simulink model "dsp48_firs_tb"  (Simulink 7.0)
settings: Solver=ode45  StartTime=0.0  StopTime=200  RelTol=1e-3
PreLoadFcn:
  | fir_setup_v1
StartFcn:
  | fir_setup_v1
undefined symbols (not defined in the file): A, B, C, coef, P, PCIN
libraries: xbsIndex_r4 x229, simulink x10, xbsCopyrightNotice_r4 x1, dspsrcs4 x1
(part 1 of 3)
settings Model: Creator=alexc  LastModifiedBy=douangp
settings DataIOCC: SignalLoggingName=sigsOut
settings OptimizationCC: InlineInvariantSignals=on
settings DebuggingCC: SaveWithParameterizedLinksMsg=none  SignalResolutionControl=TryResolveAllWithWarning  SolverPrmCheckMsg=none  MultiTaskDSMMsg=warning  MultiTaskCondExecSysMsg=none  StrictBusMsg=None
settings HardwareCC: TargetUnknown=on
settings RTWCC: IncludeERTFirstTime=on
settings GRTTargetCC: TargetFcnLib=ansi_tfl_tmw.mat

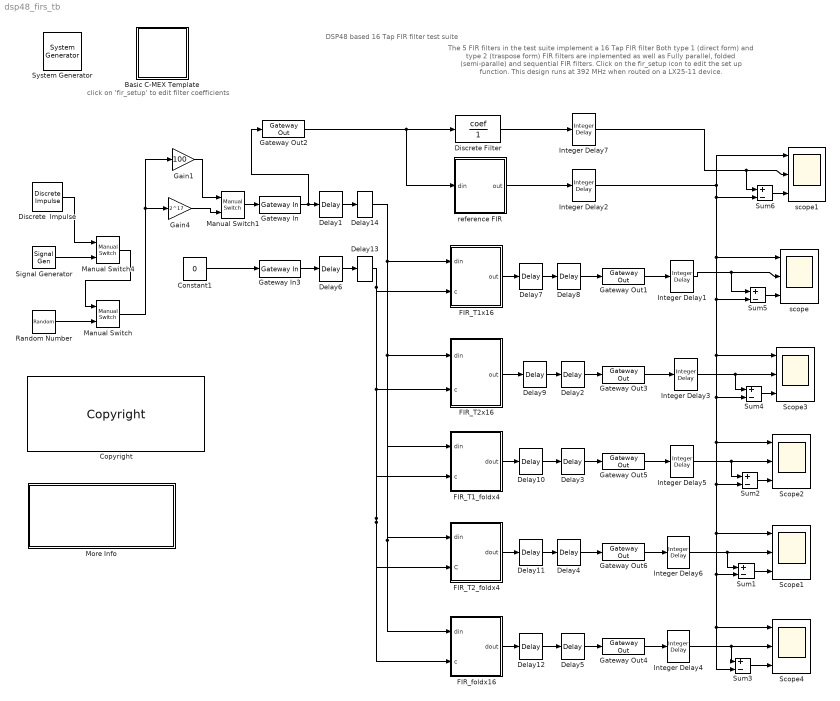
== system dsp48_firs_tb ==
  note: DSP48 based 16 Tap FIR filter test suite
  note: The 5 FIR filters in the test suite implement a 16 Tap FIR filter
      | Both type 1 (direct form) and type 2 (traspose form) FIR filters
      | are inplemented as well as Fully parallel, folded (semi-paralle)
      | and sequential FIR filters. Click on the fir_setup icon to edit the
      |  set up function.
      |
      | This design runs at 392 MHz when routed on a LX25-11 device.
  note: click on 'fir_setup'
      | to edit filter coefficients
  " System Generator" : xbsIndex_r4/ System Generator  Tag=genX  SystemSampleTime=-1  xilinxfamily=virtex4  part=xc4vlx25  speed=-11  package=ff668  synthesis_tool=XST  clock_wrapper=Clock Enables  directory=./netlist  testbench=off  simulink_period=1/16  sysclk_period=2.551  dcm_input_clock_period=100  incr_netlist=off  trim_vbits=Everywhere in SubSystem  dbl_ovrd=According to Block Masks  core_generation=According to Block Masks  run_coregen=off  deprecated_control=off  eval_field=0  block_type=system_generator
      settings: block_version=8.2.EA1
  "Basic C-MEX Template " : Subsystem  AncestorBlock=|
      | sfundemos/C-file
      | S-functions/Basic C-MEX
      | Template
      settings: OpenFcn=evalin('base','edit(''fir_setup_v1.m'')')
      mask Display:
      | plot([.8  0 0 1 1 .8 .8 1],[1 1 0 0 .7 .7 1 .7])
      | disp('fir_setup');
  Constant1 : Constant  Value=0  OutDataType=sfix(16)  OutScaling=2^0
  Copyright : xbsCopyrightNotice_r4/Copyright  block_type=copyright
      settings: block_version=10.1.00
      settings: infoedit=|
      | Copyright(C) 2008 by  Xilinx, Inc. All rights reserved.<br>
      | <br>
      | This file contains proprietary, confidential information of Xilinx, Inc., is distributed under license
      | from Xilinx, Inc., and may be used, copied and/or disclosed only pursuant to the terms of a valid license
      | agreement with Xilinx, Inc. Xilinx hereby grants you a license to use this file solely for design,
      | simulation, implementation and creation of design files limited to Xilinx devices or technologies. Use
      | with non-Xilinx devices or technologies is expressly prohibited and immediately terminates your license
      | unless covered by a separate agreement.<br>
      | <br>
      | Xilinx is providing this design, code, or information "as-is" solely for use in developing programs and
      | solutions for Xilinx devices, with no obligation on the part of Xilinx to provide support. By providing
      | this design, code, or information as one possible implementation of this feature, application or standard,
      | Xilinx is making no representation that this implementation is free from any claims of infringement. You
      | are responsible for obtaining any rights you may require for your implementation. Xilinx expressly disclaims
      | any warranty whatsoever with respect to the adequacy of the implementation, including but not limited to any
      | warranties or representations that this implementation is free from claims of infringement, implied warranties
      | of merchantability or fitness for a particular purpose.<br>
      | <br>
      | Xilinx products are not intended for use in life support appliances, devices, or systems. Use in such
      | applications is expressly prohibited.<br>
      | <br>
      | Any modifications that are made to the Source Code are done at the user's sole risk and will be unsupported.<br>
      | <br>
      | This copyright and support notice must be retained as part of this text at all times.
      | (c) Copyright 1995-2008 Xilinx, Inc. All rights reserved.
  Delay{1..14} (14 alike) : xbsIndex_r4/Delay  en=off  latency=1  dbl_ovrd=off  reg_retiming=off  block_type=delay
      settings: infoedit="Delay line having  configurable length.<P><P>Hardware notes: A delay line is a chain, each link of which is an SRL16 followed by a flip-flop. If register retiming is enabled, the delay line is a chain of flip-flops."  xl_area=[0, 0, 0, 0, 0, 0, 0]  block_version=VER_STRING_GOES_HERE
  Discrete  Impulse : dspsrcs4/Discrete  Impulse  Delay=0  SampleTime=1  FrameSample=1  dataType=double  isSigned=on  wordLen=16  udDataType=sfix(16)  fracBitsMode=Best precision  numFracBits=15
  Discrete Filter : DiscreteFilter  Numerator=coef  Denominator=1
  FIR_T1_foldx4 : Subsystem
  FIR_T1x16 : Subsystem
  FIR_T2_foldx4 : Subsystem
  "FIR_T2x16 " : Subsystem
  FIR_foldx16 : Subsystem
  Gain1 : Gain  Gain=100  ParameterDataType=sfix(16)  ParameterScaling=2^0  OutDataType=sfix(16)  OutScaling=2^0  SampleTime=1  SaturateOnIntegerOverflow=on
  Gain4 : Gain  Gain=2^17  ParameterDataType=sfix(16)  ParameterScaling=2^0  OutDataType=sfix(16)  OutScaling=2^0  SampleTime=1  SaturateOnIntegerOverflow=on
  Gateway In : xbsIndex_r4/Gateway In  arith_type="Signed  (2's comp)"  n_bits=18  bin_pt=0  quantization="Round  (unbiased: +/- Inf)"  overflow=Saturate  period=1  dbl_ovrd=off  timing_constraint=None  locs_specified=off  LOCs={}  block_type=gatewayin
      settings: infoedit="Gateway in block.  Converts inputs of type Simulink integer, double and fixed point to  Xilinx fixed point type.<P><P>Hardware notes:  In hardware these blocks become top level input ports."  xl_area=[0, 0, 0, 0, 0, 0, 0]  block_version=VER_STRING_GOES_HERE
  Gateway In3 : xbsIndex_r4/Gateway In  arith_type="Signed  (2's comp)"  n_bits=48  bin_pt=0  quantization="Round  (unbiased: +/- Inf)"  overflow=Saturate  period=1  dbl_ovrd=off  timing_constraint=None  locs_specified=off  LOCs={}  block_type=gatewayin
      settings: infoedit="Gateway in block.  Converts inputs of type Simulink integer, double and fixed point to  Xilinx fixed point type.<P><P>Hardware notes:  In hardware these blocks become top level input ports."  xl_area=[0, 0, 0, 0, 0, 0, 0]  block_version=VER_STRING_GOES_HERE
  Gateway Out{1..6} (6 alike) : xbsIndex_r4/Gateway Out  hdl_port=on  timing_constraint=None  locs_specified=off  LOCs={}  block_type=gatewayout
      settings: infoedit="Gateway out block.  Converts Xilinx fixed point inputs into ouputs of type Simulink integer, double, or fixed point.<P><P>Hardware notes:  In hardware these blocks become top level output ports or are discarded, depending on how they are configured."  xl_area=[0, 0, 0, 0, 0, 0, 0]  block_version=VER_STRING_GOES_HERE
  Integer Delay1 : simulink/Discrete/Integer Delay  vinit=0.0  samptime=-1  NumDelays=2
  Integer Delay2 : simulink/Discrete/Integer Delay  vinit=0.0  samptime=-1  NumDelays=25
  Integer Delay3 : simulink/Discrete/Integer Delay  vinit=0.0  samptime=-1  NumDelays=18
  Integer Delay4 : simulink/Discrete/Integer Delay  vinit=0.0  samptime=-1  NumDelays=17
  Integer Delay5 : simulink/Discrete/Integer Delay  vinit=0.0  samptime=-1  NumDelays=14
  Integer Delay6 : simulink/Discrete/Integer Delay  vinit=0.0  samptime=-1  NumDelays=12
  Integer Delay7 : simulink/Discrete/Integer Delay  vinit=0.0  samptime=-1  NumDelays=25
  Manual Switch : simulink/Signal Routing/Manual Switch  SystemSampleTime=-1  sw=0  action=0  varsize=off
  Manual Switch1 : simulink/Signal Routing/Manual Switch  SystemSampleTime=-1  sw=1  action=0  varsize=off
  Manual Switch4 : simulink/Signal Routing/Manual Switch  SystemSampleTime=-1  sw=1  action=0  varsize=off
  More Info : Subsystem
      settings: OpenFcn=xlDoc('-book','sysgen','-topic','Hardware Design Using System Generator/Design Styles for the DSP48/Designs that Use DSP48 and DSP48 Macro Blocks');
      mask Display: disp('Double click\n for System Generator\n documentation on related topics.')
  Random Number : RandomNumber  SampleTime=1
  Scope{1..4} (4 alike) : Scope  NumInputPorts=3
      Scope1 settings: TimeRange=200  YMin=-1e+007~-1e+007~-90  YMax=1e+007~1e+007~0
      Scope2 settings: TimeRange=200  YMin=129.2~105~105  YMax=142.8~140~140
      Scope3 settings: TimeRange=200  YMin=129.2~105~105  YMax=142.8~140~140  SaveName=ScopeData2
      Scope4 settings: TimeRange=200  YMin=-12500~-10000~950  YMax=7500~7000~1050  SaveName=ScopeData5
  Signal Generator : SignalGenerator  Frequency=.01
  Sum{1..6} (6 alike) : Sum  Inputs=+-  OutDataType=sfix(16)  OutScaling=2^0  SaturateOnIntegerOverflow=on
  reference FIR : Subsystem
  scope : Scope  NumInputPorts=3
      settings: TimeRange=200  YMin=-7500~-7500~-8000  YMax=12500~12500~7000  SaveName=ScopeData3
  scope1 : Scope  NumInputPorts=3
      settings: TimeRange=200  YMin=-12500~-12500~-1  YMax=7500~7500~1  SaveName=ScopeData4
  wires:
  Random Number/1 -> Manual Switch/2
  Gateway In/1 -> Delay1/1, Gateway Out2/1
  Constant1/1 -> Gateway In3/1
  Delay8/1 -> Gateway Out1/1
  Gateway Out1/1 -> Integer Delay1/1
  Delay2/1 -> Gateway Out3/1
  Gateway Out3/1 -> Integer Delay3/1
  Gateway Out5/1 -> Integer Delay5/1
  Gateway Out6/1 -> Integer Delay6/1
  Sum3/1 -> Scope4/3
  Manual Switch4/1 -> Manual Switch/1
  Signal Generator/1 -> Manual Switch4/2
  Discrete  Impulse/1 -> Manual Switch4/1
  FIR_T1_foldx4/1(dout) -> Delay10/1
  FIR_T2_foldx4/1(dout) -> Delay11/1
  FIR_foldx16/1(dout) -> Delay12/1
  Delay3/1 -> Gateway Out5/1
  Delay4/1 -> Gateway Out6/1
  Delay5/1 -> Gateway Out4/1
  Manual Switch/1 -> Gain4/1, Gain1/1
  Gateway In3/1 -> Delay6/1
  Delay1/1 -> Delay14/1
  Delay6/1 -> Delay13/1
  Integer Delay4/1 -> Scope4/2, Sum3/1
  Sum1/1 -> Scope1/3
  Integer Delay6/1 -> Sum1/1, Scope1/2
  Sum2/1 -> Scope2/3
  Integer Delay5/1 -> Scope2/2, Sum2/1
  Sum4/1 -> Scope3/3
  Integer Delay3/1 -> Sum4/1, Scope3/2
  Sum5/1 -> scope/3
  Integer Delay1/1 -> scope/2, Sum5/1
  reference FIR/1(out) -> Integer Delay2/1
  Integer Delay2/1 -> Scope3/1, Sum3/2, Scope4/1, Sum1/2, Scope1/1, Sum2/2, Scope2/1, Sum4/2, Sum5/2, scope/1, Sum6/2, scope1/1
  Manual Switch1/1 -> Gateway In/1
  Gain4/1 -> Manual Switch1/2
  Gain1/1 -> Manual Switch1/1
  Sum6/1 -> scope1/3
  Discrete Filter/1 -> Integer Delay7/1
  Integer Delay7/1 -> Sum6/1, scope1/2
  Gateway Out2/1 -> reference FIR/1(din), Discrete Filter/1
  Delay7/1 -> Delay8/1
  Delay9/1 -> Delay2/1
  Delay10/1 -> Delay3/1
  Delay11/1 -> Delay4/1
  Delay12/1 -> Delay5/1
  Delay13/1 -> FIR_T1_foldx4/2(c), FIR_T2_foldx4/2(C), FIR_foldx16/2(c), "FIR_T2x16 "/2(c), FIR_T1x16/2(c)
  Delay14/1 -> FIR_T1x16/1(din), FIR_T2_foldx4/1(din), FIR_T1_foldx4/1(din), FIR_foldx16/1(din), "FIR_T2x16 "/1(din)
  "FIR_T2x16 "/1(out) -> Delay9/1
  FIR_T1x16/1(out) -> Delay7/1
  Gateway Out4/1 -> Integer Delay4/1

== system dsp48_firs_tb/Basic C-MEX Template  ==
  "Basic C-MEX Template " : Subsystem  AncestorBlock=|
      | sfundemos/C-file
      | S-functions/Basic C-MEX
      | Template
      settings: OpenFcn=evalin('base','edit(''make_nio_io_cyc.m'')')
      mask Display:
      | plot([.8  0 0 1 1 .8 .8 1],[1 1 0 0 .7 .7 1 .7])
      | disp('make_nio_io_cyc.m');

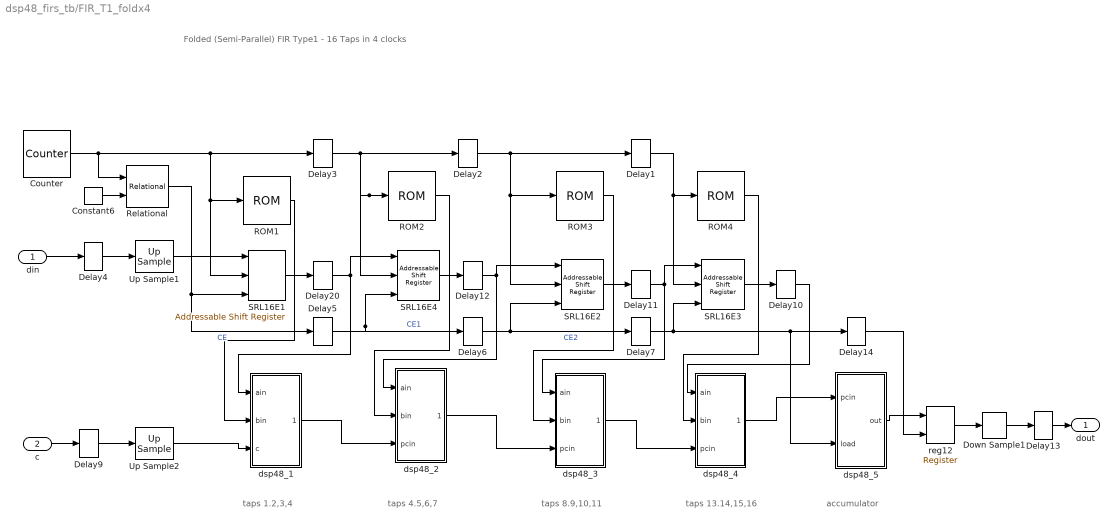
== system dsp48_firs_tb/FIR_T1_foldx4 ==
  note: Folded (Semi-Parallel) FIR Type1 - 16 Taps in 4 clocks
  note: taps 1.2,3,4
  note: taps 4.5,6,7
  note: taps 8.9,10,11
  note: taps 13.14,15,16
  note: accumulator
  din : Inport  OutDataType=sfix(16)  OutScaling=2^0
  c : Inport  Port=2  OutDataType=sfix(16)  OutScaling=2^0
  Constant6 : xbsIndex_r4/Constant  arith_type=Unsigned  const=3  n_bits=2  bin_pt=0  explicit_period=off  period=1  equ=P=C  opselect=C  inp2=PCIN>>17  opr=+  inp1=P  carry=CIN  dbl_ovrd=off  block_type=constant
      settings: block_version=VER_STRING_GOES_HERE
  Counter : xbsIndex_r4/Counter  cnt_type=Count Limited  cnt_to=3  operation=Up  start_count=0  cnt_by_val=1  arith_type=Unsigned  n_bits=2  bin_pt=0  load_pin=off  rst=off  en=off  explicit_period=off  period=1/4  dbl_ovrd=off  use_behavioral_HDL=off  use_rpm=off  block_type=counter
      settings: infoedit="Configurable up, down and up/down counter.<P><P>Hardware notes: Free running counters are the least expensive in hardware.  A count limited counter is implemented by combining a counter with a comparator."  xl_area=[2 2 0 3 0 0 0]  block_version=VER_STRING_GOES_HERE
  Delay{1..7,9..14,20} (14 alike) : xbsIndex_r4/Delay  en=off  latency=1  dbl_ovrd=off  reg_retiming=off  block_type=delay
      settings: infoedit="Delay line having  configurable length.<P><P>Hardware notes: A delay line is a chain, each link of which is an SRL16 followed by a flip-flop. If register retiming is enabled, the delay line is a chain of flip-flops."  xl_area=[0, 0, 0, 0, 0, 0, 0]  block_version=VER_STRING_GOES_HERE
  Down Sample1 : xbsIndex_r4/Down Sample  sample_ratio=4  sample_phase="Last Value of Frame  (most efficient)"  en=off  latency=1  dbl_ovrd=off  block_type=dsamp
      settings: xl_area=[24 48 0 0 0 0 0]  block_version=VER_STRING_GOES_HERE
  ROM1 : xbsIndex_r4/ROM  depth=4  initVector=coef(1:4)  distributed_mem=Distributed memory  rst=off  init_reg=0  en=off  latency=1  arith_type="Signed  (2's comp)"  n_bits=18  bin_pt=0  dbl_ovrd=off  optimize=Area  use_rpm=off  block_type=sprom
      settings: xl_area=[0, 0, 0, 0, 0, 0, 0]  block_version=VER_STRING_GOES_HERE
  ROM2 : xbsIndex_r4/ROM  depth=4  initVector=coef(5:8)  distributed_mem=Distributed memory  rst=off  init_reg=0  en=off  latency=1  arith_type="Signed  (2's comp)"  n_bits=18  bin_pt=0  dbl_ovrd=off  optimize=Area  use_rpm=off  block_type=sprom
      settings: xl_area=[0, 0, 0, 0, 0, 0, 0]  block_version=VER_STRING_GOES_HERE
  ROM3 : xbsIndex_r4/ROM  depth=4  initVector=coef(9:12)  distributed_mem=Distributed memory  rst=off  init_reg=0  en=off  latency=1  arith_type="Signed  (2's comp)"  n_bits=18  bin_pt=0  dbl_ovrd=off  optimize=Area  use_rpm=off  block_type=sprom
      settings: xl_area=[0, 0, 0, 0, 0, 0, 0]  block_version=VER_STRING_GOES_HERE
  ROM4 : xbsIndex_r4/ROM  depth=4  initVector=coef(13:16)  distributed_mem=Distributed memory  rst=off  init_reg=0  en=off  latency=1  arith_type="Signed  (2's comp)"  n_bits=18  bin_pt=0  dbl_ovrd=off  optimize=Area  use_rpm=off  block_type=sprom
      settings: xl_area=[0, 0, 0, 0, 0, 0, 0]  block_version=VER_STRING_GOES_HERE
  Relational : xbsIndex_r4/Relational  mode=a=b  en=off  latency=0  dbl_ovrd=off  block_type=relational
      settings: xl_area=[1 0 0 1 0 0 0]  block_version=VER_STRING_GOES_HERE
  SRL16E{1..4} (4 alike) : xbsIndex_r4/Addressable Shift Register  infer_latency=off  depth=4  initVector=[0]  en=on  dbl_ovrd=off  use_behavioral_HDL=off  use_rpm=off  block_type=addrsr
      settings: infoedit="Delay of configurable length.  Any element in the delay line can be addressed and driven onto the output port.<P><P>Hardware notes: Implemented using SRL16s.  If a Virtex-II device is used, multiple SRLC16s are cascaded together."  xl_area=[9 0 0 18 0 0 0]  block_version=VER_STRING_GOES_HERE
  Up Sample1 : xbsIndex_r4/Up Sample  sample_ratio=4  copy_samples=on  dbl_ovrd=off  block_type=usamp
      settings: infoedit="Up samples input data.  Inserted values  can be zeros or copies of the most recent input sample.<P><P>Hardware notes: No hardware is needed if inserted values are copies of the input sample; otherwise, a mux and single bit flip-flop are used."  xl_area=[0 0 0 0 0 0 0]  block_version=VER_STRING_GOES_HERE
  Up Sample2 : xbsIndex_r4/Up Sample  sample_ratio=4  copy_samples=on  dbl_ovrd=off  block_type=usamp
      settings: infoedit="Up samples input data.  Inserted values  can be zeros or copies of the most recent input sample.<P><P>Hardware notes: No hardware is needed if inserted values are copies of the input sample; otherwise, a mux and single bit flip-flop are used."  xl_area=[0 0 0 0 0 0 0]  block_version=VER_STRING_GOES_HERE
  dsp48_1 : Subsystem
  dsp48_2 : Subsystem
  dsp48_3 : Subsystem
  dsp48_4 : Subsystem
  dsp48_5 : Subsystem
  reg12 : xbsIndex_r4/Register  init=0  rst=off  en=on  dbl_ovrd=off  block_type=register
      settings: xl_area=[24 48 0 0 0 0 0]  block_version=VER_STRING_GOES_HERE
  dout : Outport  OutDataType=sfix(16)  OutScaling=2^0
  wires:
  SRL16E1/1 -> Delay20/1
  SRL16E4/1 -> Delay12/1
  ROM2/1 -> dsp48_2/2(bin)
  ROM1/1 -> dsp48_1/2(bin)
  ROM3/1 -> dsp48_3/2(bin)
  ROM4/1 -> dsp48_4/2(bin)
  dsp48_2/1(pcout) -> dsp48_3/3(pcin)
  dsp48_3/1(pcout) -> dsp48_4/3(pcin)
  SRL16E2/1 -> Delay11/1
  SRL16E3/1 -> Delay10/1
  Delay2/1 -> SRL16E2/2, ROM3/1, Delay1/1
  Delay1/1 -> SRL16E3/2, ROM4/1
  Delay12/1 -> SRL16E2/1, dsp48_2/1(ain)
  Constant6/1 -> Relational/2
  din/1 -> Delay4/1
  dsp48_5/1(out) -> reg12/1
  Up Sample1/1 -> SRL16E1/1
  reg12/1 -> Down Sample1/1
  Down Sample1/1 -> Delay13/1
  Delay10/1 -> dsp48_4/1(ain)
  Delay3/1 -> Delay2/1, SRL16E4/2, ROM2/1
  Delay20/1 -> dsp48_1/1(ain), SRL16E4/1
  Up Sample2/1 -> dsp48_1/3(c)
  c/1 -> Delay9/1
  Delay11/1 -> SRL16E3/1, dsp48_3/1(ain)
  dsp48_4/1(pcout) -> dsp48_5/1(pcin)
  Counter/1 -> Relational/1, ROM1/1, SRL16E1/2, Delay3/1
  Relational/1 -> SRL16E1/3, Delay5/1  "CE"
  Delay4/1 -> Up Sample1/1
  Delay9/1 -> Up Sample2/1
  Delay13/1 -> dout/1
  dsp48_1/1(pcout) -> dsp48_2/3(pcin)
  Delay7/1 -> SRL16E3/3, dsp48_5/2(load), Delay14/1
  Delay6/1 -> Delay7/1, SRL16E2/3  "CE2"
  Delay5/1 -> Delay6/1, SRL16E4/3  "CE1"
  Delay14/1 -> reg12/2

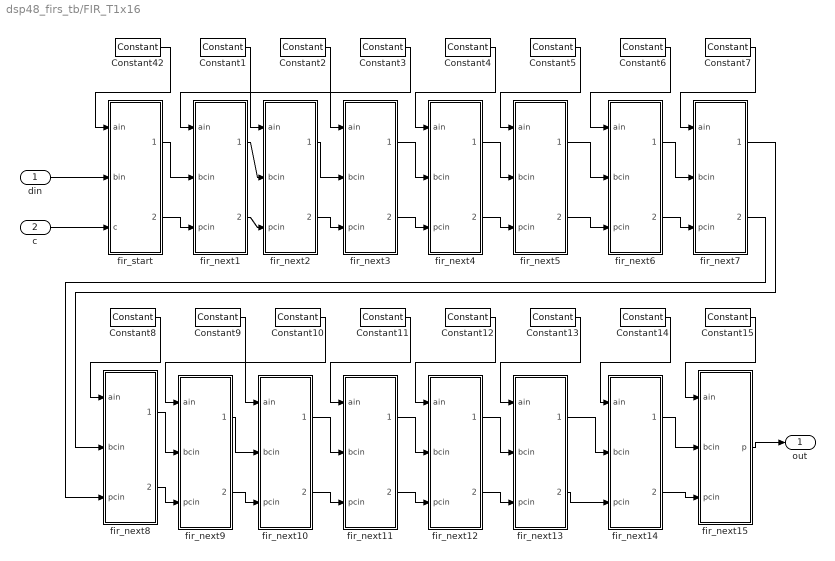
== system dsp48_firs_tb/FIR_T1x16 ==
  din : Inport  OutDataType=sfix(16)  OutScaling=2^0
  c : Inport  Port=2  OutDataType=sfix(16)  OutScaling=2^0
  Constant1 : xbsIndex_r4/Constant  arith_type=Signed (2's comp)  const=coef(2)  n_bits=18  bin_pt=0  explicit_period=off  period=1  equ=P=C  opselect=C  inp2=PCIN>>17  opr=+  inp1=P  carry=CIN  dbl_ovrd=off  block_type=constant
      settings: block_version=VER_STRING_GOES_HERE
  Constant10 : xbsIndex_r4/Constant  arith_type=Signed (2's comp)  const=coef(11)  n_bits=18  bin_pt=0  explicit_period=off  period=1  equ=P=C  opselect=C  inp2=PCIN>>17  opr=+  inp1=P  carry=CIN  dbl_ovrd=off  block_type=constant
      settings: block_version=VER_STRING_GOES_HERE
  Constant11 : xbsIndex_r4/Constant  arith_type=Signed (2's comp)  const=coef(12)  n_bits=18  bin_pt=0  explicit_period=off  period=1  equ=P=C  opselect=C  inp2=PCIN>>17  opr=+  inp1=P  carry=CIN  dbl_ovrd=off  block_type=constant
      settings: block_version=VER_STRING_GOES_HERE
  Constant12 : xbsIndex_r4/Constant  arith_type=Signed (2's comp)  const=coef(13)  n_bits=18  bin_pt=0  explicit_period=off  period=1  equ=P=C  opselect=C  inp2=PCIN>>17  opr=+  inp1=P  carry=CIN  dbl_ovrd=off  block_type=constant
      settings: block_version=VER_STRING_GOES_HERE
  Constant13 : xbsIndex_r4/Constant  arith_type=Signed (2's comp)  const=coef(14)  n_bits=18  bin_pt=0  explicit_period=off  period=1  equ=P=C  opselect=C  inp2=PCIN>>17  opr=+  inp1=P  carry=CIN  dbl_ovrd=off  block_type=constant
      settings: block_version=VER_STRING_GOES_HERE
  Constant14 : xbsIndex_r4/Constant  arith_type=Signed (2's comp)  const=coef(15)  n_bits=18  bin_pt=0  explicit_period=off  period=1  equ=P=C  opselect=C  inp2=PCIN>>17  opr=+  inp1=P  carry=CIN  dbl_ovrd=off  block_type=constant
      settings: block_version=VER_STRING_GOES_HERE
  Constant15 : xbsIndex_r4/Constant  arith_type=Signed (2's comp)  const=coef(16)  n_bits=18  bin_pt=0  explicit_period=off  period=1  equ=P=C  opselect=C  inp2=PCIN>>17  opr=+  inp1=P  carry=CIN  dbl_ovrd=off  block_type=constant
      settings: block_version=VER_STRING_GOES_HERE
  Constant2 : xbsIndex_r4/Constant  arith_type=Signed (2's comp)  const=coef(3)  n_bits=18  bin_pt=0  explicit_period=off  period=1  equ=P=C  opselect=C  inp2=PCIN>>17  opr=+  inp1=P  carry=CIN  dbl_ovrd=off  block_type=constant
      settings: block_version=VER_STRING_GOES_HERE
  Constant3 : xbsIndex_r4/Constant  arith_type=Signed (2's comp)  const=coef(4)  n_bits=18  bin_pt=0  explicit_period=off  period=1  equ=P=C  opselect=C  inp2=PCIN>>17  opr=+  inp1=P  carry=CIN  dbl_ovrd=off  block_type=constant
      settings: block_version=VER_STRING_GOES_HERE
  Constant4 : xbsIndex_r4/Constant  arith_type=Signed (2's comp)  const=coef(5)  n_bits=18  bin_pt=0  explicit_period=off  period=1  equ=P=C  opselect=C  inp2=PCIN>>17  opr=+  inp1=P  carry=CIN  dbl_ovrd=off  block_type=constant
      settings: block_version=VER_STRING_GOES_HERE
  Constant42 : xbsIndex_r4/Constant  arith_type=Signed (2's comp)  const=coef(1)  n_bits=18  bin_pt=0  explicit_period=off  period=1  equ=P=C  opselect=C  inp2=PCIN>>17  opr=+  inp1=P  carry=CIN  dbl_ovrd=off  block_type=constant
      settings: block_version=VER_STRING_GOES_HERE
  Constant5 : xbsIndex_r4/Constant  arith_type=Signed (2's comp)  const=coef(6)  n_bits=18  bin_pt=0  explicit_period=off  period=1  equ=P=C  opselect=C  inp2=PCIN>>17  opr=+  inp1=P  carry=CIN  dbl_ovrd=off  block_type=constant
      settings: block_version=VER_STRING_GOES_HERE
  Constant6 : xbsIndex_r4/Constant  arith_type=Signed (2's comp)  const=coef(7)  n_bits=18  bin_pt=0  explicit_period=off  period=1  equ=P=C  opselect=C  inp2=PCIN>>17  opr=+  inp1=P  carry=CIN  dbl_ovrd=off  block_type=constant
      settings: block_version=VER_STRING_GOES_HERE
  Constant7 : xbsIndex_r4/Constant  arith_type=Signed (2's comp)  const=coef(8)  n_bits=18  bin_pt=0  explicit_period=off  period=1  equ=P=C  opselect=C  inp2=PCIN>>17  opr=+  inp1=P  carry=CIN  dbl_ovrd=off  block_type=constant
      settings: block_version=VER_STRING_GOES_HERE
  Constant8 : xbsIndex_r4/Constant  arith_type=Signed (2's comp)  const=coef(9)  n_bits=18  bin_pt=0  explicit_period=off  period=1  equ=P=C  opselect=C  inp2=PCIN>>17  opr=+  inp1=P  carry=CIN  dbl_ovrd=off  block_type=constant
      settings: block_version=VER_STRING_GOES_HERE
  Constant9 : xbsIndex_r4/Constant  arith_type=Signed (2's comp)  const=coef(10)  n_bits=18  bin_pt=0  explicit_period=off  period=1  equ=P=C  opselect=C  inp2=PCIN>>17  opr=+  inp1=P  carry=CIN  dbl_ovrd=off  block_type=constant
      settings: block_version=VER_STRING_GOES_HERE
  fir_next1 : Subsystem
  fir_next10 : Subsystem
  fir_next11 : Subsystem
  fir_next12 : Subsystem
  fir_next13 : Subsystem
  fir_next14 : Subsystem
  fir_next15 : Subsystem
  fir_next2 : Subsystem
  fir_next3 : Subsystem
  fir_next4 : Subsystem
  fir_next5 : Subsystem
  fir_next6 : Subsystem
  fir_next7 : Subsystem
  fir_next8 : Subsystem
  fir_next9 : Subsystem
  fir_start : Subsystem
  out : Outport  OutDataType=sfix(16)  OutScaling=2^0
  wires:
  fir_next15/1(p) -> out/1
  Constant15/1 -> fir_next15/1(ain)
  fir_next14/1(bcout) -> fir_next15/2(bcin)
  fir_next14/2(pcout) -> fir_next15/3(pcin)
  Constant14/1 -> fir_next14/1(ain)
  fir_next13/1(bcout) -> fir_next14/2(bcin)
  fir_next13/2(pcout) -> fir_next14/3(pcin)
  Constant13/1 -> fir_next13/1(ain)
  fir_next12/1(bcout) -> fir_next13/2(bcin)
  fir_next12/2(pcout) -> fir_next13/3(pcin)
  Constant12/1 -> fir_next12/1(ain)
  fir_next11/1(bcout) -> fir_next12/2(bcin)
  fir_next11/2(pcout) -> fir_next12/3(pcin)
  Constant11/1 -> fir_next11/1(ain)
  fir_next10/1(bcout) -> fir_next11/2(bcin)
  fir_next10/2(pcout) -> fir_next11/3(pcin)
  Constant10/1 -> fir_next10/1(ain)
  fir_next9/1(bcout) -> fir_next10/2(bcin)
  fir_next9/2(pcout) -> fir_next10/3(pcin)
  Constant9/1 -> fir_next9/1(ain)
  fir_next8/1(bcout) -> fir_next9/2(bcin)
  fir_next8/2(pcout) -> fir_next9/3(pcin)
  Constant8/1 -> fir_next8/1(ain)
  fir_next7/1(bcout) -> fir_next8/2(bcin)
  fir_next7/2(pcout) -> fir_next8/3(pcin)
  Constant7/1 -> fir_next7/1(ain)
  fir_next6/1(bcout) -> fir_next7/2(bcin)
  fir_next6/2(pcout) -> fir_next7/3(pcin)
  Constant6/1 -> fir_next6/1(ain)
  fir_next5/1(bcout) -> fir_next6/2(bcin)
  fir_next5/2(pcout) -> fir_next6/3(pcin)
  Constant5/1 -> fir_next5/1(ain)
  fir_next4/1(bcout) -> fir_next5/2(bcin)
  fir_next4/2(pcout) -> fir_next5/3(pcin)
  Constant4/1 -> fir_next4/1(ain)
  fir_next3/1(bcout) -> fir_next4/2(bcin)
  fir_next3/2(pcout) -> fir_next4/3(pcin)
  Constant3/1 -> fir_next3/1(ain)
  fir_next2/1(bcout) -> fir_next3/2(bcin)
  fir_next2/2(pcout) -> fir_next3/3(pcin)
  Constant2/1 -> fir_next2/1(ain)
  fir_next1/1(bcout) -> fir_next2/2(bcin)
  fir_next1/2(pcout) -> fir_next2/3(pcin)
  Constant1/1 -> fir_next1/1(ain)
  Constant42/1 -> fir_start/1(ain)
  fir_start/1(bcout) -> fir_next1/2(bcin)
  c/1 -> fir_start/3(c)
  din/1 -> fir_start/2(bin)
  fir_start/2(pcout) -> fir_next1/3(pcin)

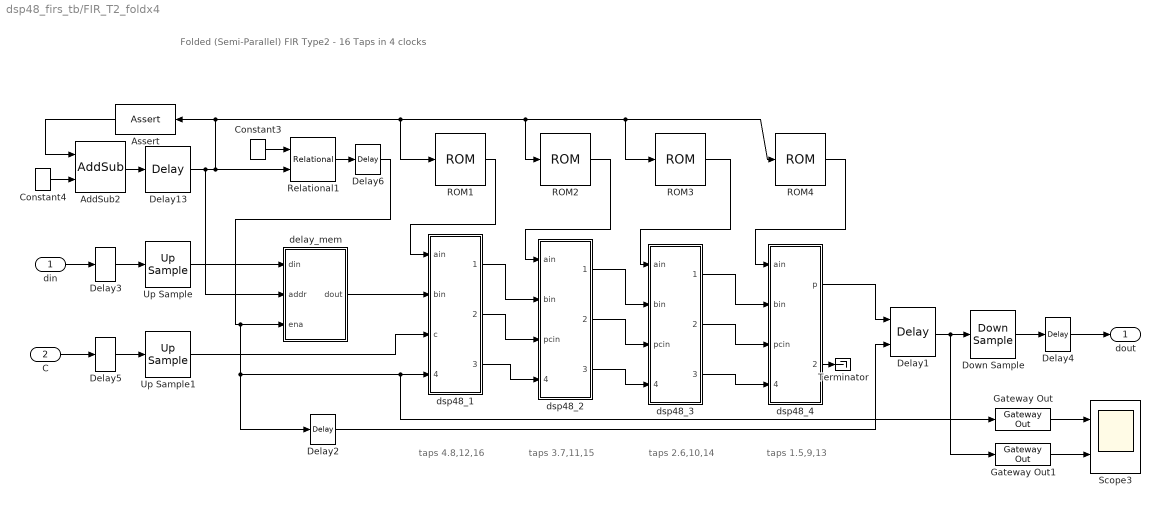
== system dsp48_firs_tb/FIR_T2_foldx4 ==
  note: Folded (Semi-Parallel) FIR Type2 - 16 Taps in 4 clocks
  note: taps 4.8,12,16
  note: taps 3.7,11,15
  note: taps 2.6,10,14
  note: taps 1.5,9,13
  din : Inport  OutDataType=sfix(16)  OutScaling=2^0
  C : Inport  Port=2  OutDataType=sfix(16)  OutScaling=2^0
  AddSub2 : xbsIndex_r4/AddSub  mode=Addition  use_carryin=off  use_carryout=off  en=off  latency=0  precision=User Defined  arith_type=Unsigned  n_bits=2  bin_pt=0  quantization=Truncate  overflow=Wrap  dbl_ovrd=off  use_behavioral_HDL=off  pipelined=off  use_rpm=off  block_type=addsub
      settings: xl_area=[0, 0, 0, 0, 0, 0, 0]  block_version=VER_STRING_GOES_HERE
  Assert : xbsIndex_r4/Assert  Orientation=left  assert_type=off  type_source=Explicitly  arith_type=Unsigned  n_bits=8  bin_pt=2  assert_rate=on  rate_source=Explicitly  period=1/4  output_port=on  block_type=assert
      settings: infoedit=Asserts a user-defined sample rate and/or type on a signal.  block_version=VER_STRING_GOES_HERE
  Constant3 : xbsIndex_r4/Constant  arith_type=Unsigned  const=2  n_bits=2  bin_pt=0  explicit_period=off  period=1  equ=P=C  opselect=C  inp2=PCIN>>17  opr=+  inp1=P  carry=CIN  dbl_ovrd=off  block_type=constant
      settings: block_version=VER_STRING_GOES_HERE
  Constant4 : xbsIndex_r4/Constant  arith_type=Unsigned  const=1  n_bits=2  bin_pt=0  explicit_period=off  period=1  equ=P=C  opselect=C  inp2=PCIN>>17  opr=+  inp1=P  carry=CIN  dbl_ovrd=off  block_type=constant
      settings: block_version=VER_STRING_GOES_HERE
  Delay1 : xbsIndex_r4/Delay  en=on  latency=1  dbl_ovrd=off  reg_retiming=off  block_type=delay
      settings: infoedit="Delay line having  configurable length.<P><P>Hardware notes: A delay line is a chain, each link of which is an SRL16 followed by a flip-flop. If register retiming is enabled, the delay line is a chain of flip-flops."  xl_area=[0, 0, 0, 0, 0, 0, 0]  block_version=VER_STRING_GOES_HERE
  Delay{2..6,13} (6 alike) : xbsIndex_r4/Delay  en=off  latency=1  dbl_ovrd=off  reg_retiming=off  block_type=delay
      settings: infoedit="Delay line having  configurable length.<P><P>Hardware notes: A delay line is a chain, each link of which is an SRL16 followed by a flip-flop. If register retiming is enabled, the delay line is a chain of flip-flops."  xl_area=[0, 0, 0, 0, 0, 0, 0]  block_version=VER_STRING_GOES_HERE
  Down Sample : xbsIndex_r4/Down Sample  sample_ratio=4  sample_phase="Last Value of Frame  (most efficient)"  en=off  latency=1  dbl_ovrd=off  block_type=dsamp
      settings: xl_area=[0, 0, 0, 0, 0, 0, 0]  block_version=VER_STRING_GOES_HERE
  Gateway Out : xbsIndex_r4/Gateway Out  hdl_port=off  timing_constraint=None  locs_specified=off  LOCs={}  block_type=gatewayout
      settings: infoedit="Gateway out block.  Converts Xilinx fixed point inputs into ouputs of type Simulink integer, double, or fixed point.<P><P>Hardware notes:  In hardware these blocks become top level output ports or are discarded, depending on how they are configured."  xl_area=[0, 0, 0, 0, 0, 0, 0]  block_version=VER_STRING_GOES_HERE
  Gateway Out1 : xbsIndex_r4/Gateway Out  hdl_port=off  timing_constraint=None  locs_specified=off  LOCs={}  block_type=gatewayout
      settings: infoedit="Gateway out block.  Converts Xilinx fixed point inputs into ouputs of type Simulink integer, double, or fixed point.<P><P>Hardware notes:  In hardware these blocks become top level output ports or are discarded, depending on how they are configured."  xl_area=[0, 0, 0, 0, 0, 0, 0]  block_version=VER_STRING_GOES_HERE
  ROM1 : xbsIndex_r4/ROM  depth=4  initVector=coef(4:4:16)  distributed_mem=Distributed memory  rst=off  init_reg=0  en=off  latency=2  arith_type="Signed  (2's comp)"  n_bits=18  bin_pt=0  dbl_ovrd=off  optimize=Area  use_rpm=off  block_type=sprom
      settings: xl_area=[0, 0, 0, 0, 0, 0, 0]  block_version=VER_STRING_GOES_HERE
  ROM2 : xbsIndex_r4/ROM  depth=4  initVector=coef(3:4:15)  distributed_mem=Distributed memory  rst=off  init_reg=0  en=off  latency=2  arith_type="Signed  (2's comp)"  n_bits=18  bin_pt=0  dbl_ovrd=off  optimize=Area  use_rpm=off  block_type=sprom
      settings: xl_area=[0, 0, 0, 0, 0, 0, 0]  block_version=VER_STRING_GOES_HERE
  ROM3 : xbsIndex_r4/ROM  depth=4  initVector=coef(2:4:14)  distributed_mem=Distributed memory  rst=off  init_reg=0  en=off  latency=2  arith_type="Signed  (2's comp)"  n_bits=18  bin_pt=0  dbl_ovrd=off  optimize=Area  use_rpm=off  block_type=sprom
      settings: xl_area=[0, 0, 0, 0, 0, 0, 0]  block_version=VER_STRING_GOES_HERE
  ROM4 : xbsIndex_r4/ROM  depth=4  initVector=coef(1:4:13)  distributed_mem=Distributed memory  rst=off  init_reg=0  en=off  latency=2  arith_type="Signed  (2's comp)"  n_bits=18  bin_pt=0  dbl_ovrd=off  optimize=Area  use_rpm=off  block_type=sprom
      settings: xl_area=[0, 0, 0, 0, 0, 0, 0]  block_version=VER_STRING_GOES_HERE
  Relational1 : xbsIndex_r4/Relational  mode=a=b  en=off  latency=0  dbl_ovrd=off  block_type=relational
      settings: xl_area=[0, 0, 0, 0, 0, 0, 0]  block_version=VER_STRING_GOES_HERE
  Scope3 : Scope  NumInputPorts=2
      settings: TimeRange=200  YMin=0~-4000  YMax=1~3500  SaveName=ScopeData6
  Terminator : Terminator
  Up Sample : xbsIndex_r4/Up Sample  sample_ratio=4  copy_samples=on  dbl_ovrd=off  block_type=usamp
      settings: infoedit="Up samples input data.  Inserted values  can be zeros or copies of the most recent input sample.<P><P>Hardware notes: No hardware is needed if inserted values are copies of the input sample; otherwise, a mux and single bit flip-flop are used."  xl_area=[0, 0, 0, 0, 0, 0, 0]  block_version=VER_STRING_GOES_HERE
  Up Sample1 : xbsIndex_r4/Up Sample  sample_ratio=4  copy_samples=on  dbl_ovrd=off  block_type=usamp
      settings: infoedit="Up samples input data.  Inserted values  can be zeros or copies of the most recent input sample.<P><P>Hardware notes: No hardware is needed if inserted values are copies of the input sample; otherwise, a mux and single bit flip-flop are used."  xl_area=[0, 0, 0, 0, 0, 0, 0]  block_version=VER_STRING_GOES_HERE
  delay_mem : Subsystem
  dsp48_1 : Subsystem
  dsp48_2 : Subsystem
  dsp48_3 : Subsystem
  dsp48_4 : Subsystem
  dout : Outport  OutDataType=sfix(16)  OutScaling=2^0
  wires:
  AddSub2/1 -> Delay13/1
  Constant4/1 -> AddSub2/2
  Delay2/1 -> Delay1/2
  Down Sample/1 -> Delay4/1
  din/1 -> Delay3/1
  Up Sample/1 -> delay_mem/1(din)
  Constant3/1 -> Relational1/1
  Delay3/1 -> Up Sample/1
  Delay4/1 -> dout/1
  delay_mem/1(dout) -> dsp48_1/2(bin)
  ROM1/1 -> dsp48_1/1(ain)
  ROM2/1 -> dsp48_2/1(ain)
  ROM3/1 -> dsp48_3/1(ain)
  ROM4/1 -> dsp48_4/1(ain)
  Delay1/1 -> Down Sample/1, Gateway Out1/1
  dsp48_1/1(bout) -> dsp48_2/2(bin)
  dsp48_1/2(pcout) -> dsp48_2/3(pcin)
  dsp48_1/3(loado) -> dsp48_2/4(load)
  dsp48_2/1(bout) -> dsp48_3/2(bin)
  dsp48_3/1(bout) -> dsp48_4/2(bin)
  dsp48_3/2(pcout) -> dsp48_4/3(pcin)
  dsp48_3/3(loado) -> dsp48_4/4(load)
  dsp48_2/2(pcout) -> dsp48_3/3(pcin)
  dsp48_2/3(loado) -> dsp48_3/4(load)
  dsp48_4/1(p) -> Delay1/1
  Relational1/1 -> Delay6/1
  C/1 -> Delay5/1
  Delay13/1 -> Relational1/2, ROM4/1, ROM3/1, ROM2/1, ROM1/1, Assert/1, delay_mem/2(addr)
  Up Sample1/1 -> dsp48_1/3(c)
  Delay5/1 -> Up Sample1/1
  Delay6/1 -> delay_mem/3(ena), Delay2/1, dsp48_1/4(load), Gateway Out/1
  Gateway Out/1 -> Scope3/1
  Gateway Out1/1 -> Scope3/2
  Assert/1 -> AddSub2/1
  dsp48_4/2(loado) -> Terminator/1

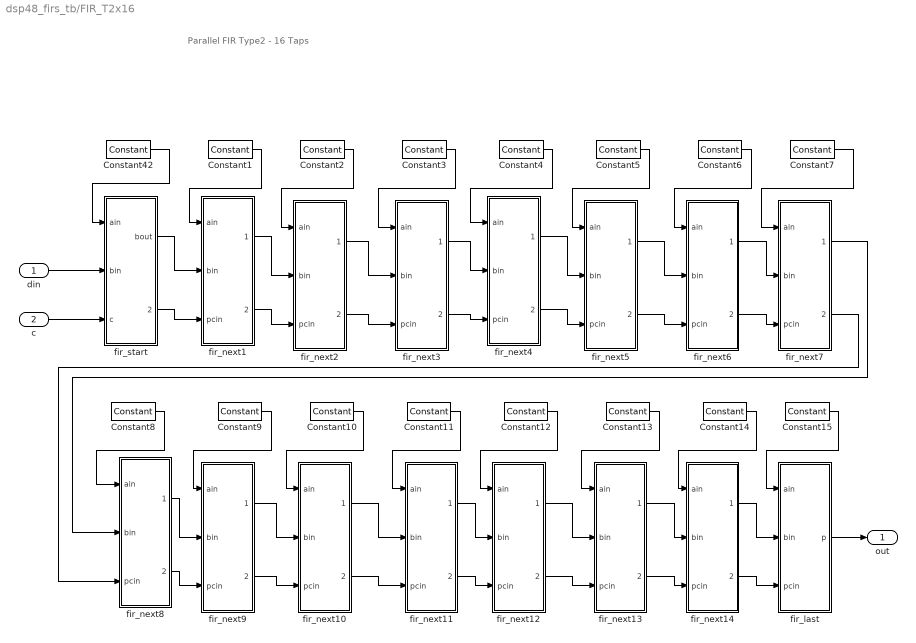
== system dsp48_firs_tb/FIR_T2x16  ==
  note: Parallel FIR Type2 - 16 Taps
  din : Inport  OutDataType=sfix(16)  OutScaling=2^0
  c : Inport  Port=2  OutDataType=sfix(16)  OutScaling=2^0
  Constant1 : xbsIndex_r4/Constant  arith_type=Signed (2's comp)  const=coef(15)  n_bits=18  bin_pt=0  explicit_period=off  period=1  equ=P=C  opselect=C  inp2=PCIN>>17  opr=+  inp1=P  carry=CIN  dbl_ovrd=off  block_type=constant
      settings: block_version=VER_STRING_GOES_HERE
  Constant10 : xbsIndex_r4/Constant  arith_type=Signed (2's comp)  const=coef(6)  n_bits=18  bin_pt=0  explicit_period=off  period=1  equ=P=C  opselect=C  inp2=PCIN>>17  opr=+  inp1=P  carry=CIN  dbl_ovrd=off  block_type=constant
      settings: block_version=VER_STRING_GOES_HERE
  Constant11 : xbsIndex_r4/Constant  arith_type=Signed (2's comp)  const=coef(5)  n_bits=18  bin_pt=0  explicit_period=off  period=1  equ=P=C  opselect=C  inp2=PCIN>>17  opr=+  inp1=P  carry=CIN  dbl_ovrd=off  block_type=constant
      settings: block_version=VER_STRING_GOES_HERE
  Constant12 : xbsIndex_r4/Constant  arith_type=Signed (2's comp)  const=coef(4)  n_bits=18  bin_pt=0  explicit_period=off  period=1  equ=P=C  opselect=C  inp2=PCIN>>17  opr=+  inp1=P  carry=CIN  dbl_ovrd=off  block_type=constant
      settings: block_version=VER_STRING_GOES_HERE
  Constant13 : xbsIndex_r4/Constant  arith_type=Signed (2's comp)  const=coef(3)  n_bits=18  bin_pt=0  explicit_period=off  period=1  equ=P=C  opselect=C  inp2=PCIN>>17  opr=+  inp1=P  carry=CIN  dbl_ovrd=off  block_type=constant
      settings: block_version=VER_STRING_GOES_HERE
  Constant14 : xbsIndex_r4/Constant  arith_type=Signed (2's comp)  const=coef(2)  n_bits=18  bin_pt=0  explicit_period=off  period=1  equ=P=C  opselect=C  inp2=PCIN>>17  opr=+  inp1=P  carry=CIN  dbl_ovrd=off  block_type=constant
      settings: block_version=VER_STRING_GOES_HERE
  Constant15 : xbsIndex_r4/Constant  arith_type=Signed (2's comp)  const=coef(1)  n_bits=18  bin_pt=0  explicit_period=off  period=1  equ=P=C  opselect=C  inp2=PCIN>>17  opr=+  inp1=P  carry=CIN  dbl_ovrd=off  block_type=constant
      settings: block_version=VER_STRING_GOES_HERE
  Constant2 : xbsIndex_r4/Constant  arith_type=Signed (2's comp)  const=coef(14)  n_bits=18  bin_pt=0  explicit_period=off  period=1  equ=P=C  opselect=C  inp2=PCIN>>17  opr=+  inp1=P  carry=CIN  dbl_ovrd=off  block_type=constant
      settings: block_version=VER_STRING_GOES_HERE
  Constant3 : xbsIndex_r4/Constant  arith_type=Signed (2's comp)  const=coef(13)  n_bits=18  bin_pt=0  explicit_period=off  period=1  equ=P=C  opselect=C  inp2=PCIN>>17  opr=+  inp1=P  carry=CIN  dbl_ovrd=off  block_type=constant
      settings: block_version=VER_STRING_GOES_HERE
  Constant4 : xbsIndex_r4/Constant  arith_type=Signed (2's comp)  const=coef(12)  n_bits=18  bin_pt=0  explicit_period=off  period=1  equ=P=C  opselect=C  inp2=PCIN>>17  opr=+  inp1=P  carry=CIN  dbl_ovrd=off  block_type=constant
      settings: block_version=VER_STRING_GOES_HERE
  Constant42 : xbsIndex_r4/Constant  arith_type=Signed (2's comp)  const=coef(16)  n_bits=18  bin_pt=0  explicit_period=off  period=1  equ=P=C  opselect=C  inp2=PCIN>>17  opr=+  inp1=P  carry=CIN  dbl_ovrd=off  block_type=constant
      settings: block_version=VER_STRING_GOES_HERE
  Constant5 : xbsIndex_r4/Constant  arith_type=Signed (2's comp)  const=coef(11)  n_bits=18  bin_pt=0  explicit_period=off  period=1  equ=P=C  opselect=C  inp2=PCIN>>17  opr=+  inp1=P  carry=CIN  dbl_ovrd=off  block_type=constant
      settings: block_version=VER_STRING_GOES_HERE
  Constant6 : xbsIndex_r4/Constant  arith_type=Signed (2's comp)  const=coef(10)  n_bits=18  bin_pt=0  explicit_period=off  period=1  equ=P=C  opselect=C  inp2=PCIN>>17  opr=+  inp1=P  carry=CIN  dbl_ovrd=off  block_type=constant
      settings: block_version=VER_STRING_GOES_HERE
  Constant7 : xbsIndex_r4/Constant  arith_type=Signed (2's comp)  const=coef(9)  n_bits=18  bin_pt=0  explicit_period=off  period=1  equ=P=C  opselect=C  inp2=PCIN>>17  opr=+  inp1=P  carry=CIN  dbl_ovrd=off  block_type=constant
      settings: block_version=VER_STRING_GOES_HERE
  Constant8 : xbsIndex_r4/Constant  arith_type=Signed (2's comp)  const=coef(8)  n_bits=18  bin_pt=0  explicit_period=off  period=1  equ=P=C  opselect=C  inp2=PCIN>>17  opr=+  inp1=P  carry=CIN  dbl_ovrd=off  block_type=constant
      settings: block_version=VER_STRING_GOES_HERE
  Constant9 : xbsIndex_r4/Constant  arith_type=Signed (2's comp)  const=coef(7)  n_bits=18  bin_pt=0  explicit_period=off  period=1  equ=P=C  opselect=C  inp2=PCIN>>17  opr=+  inp1=P  carry=CIN  dbl_ovrd=off  block_type=constant
      settings: block_version=VER_STRING_GOES_HERE
  fir_last : Subsystem
  fir_next1 : Subsystem
  fir_next10 : Subsystem
  fir_next11 : Subsystem
  fir_next12 : Subsystem
  fir_next13 : Subsystem
  fir_next14 : Subsystem
  fir_next2 : Subsystem
  fir_next3 : Subsystem
  fir_next4 : Subsystem
  fir_next5 : Subsystem
  fir_next6 : Subsystem
  fir_next7 : Subsystem
  fir_next8 : Subsystem
  fir_next9 : Subsystem
  fir_start : Subsystem
  out : Outport  OutDataType=sfix(16)  OutScaling=2^0
  wires:
  fir_next14/1(bout) -> fir_last/2(bin)
  fir_next14/2(pcout) -> fir_last/3(pcin)
  Constant15/1 -> fir_last/1(ain)
  fir_next12/2(pcout) -> fir_next13/3(pcin)
  fir_next12/1(bout) -> fir_next13/2(bin)
  fir_next13/2(pcout) -> fir_next14/3(pcin)
  fir_next13/1(bout) -> fir_next14/2(bin)
  Constant14/1 -> fir_next14/1(ain)
  Constant13/1 -> fir_next13/1(ain)
  fir_next11/2(pcout) -> fir_next12/3(pcin)
  fir_next11/1(bout) -> fir_next12/2(bin)
  Constant12/1 -> fir_next12/1(ain)
  fir_next9/2(pcout) -> fir_next10/3(pcin)
  fir_next9/1(bout) -> fir_next10/2(bin)
  fir_next10/2(pcout) -> fir_next11/3(pcin)
  fir_next10/1(bout) -> fir_next11/2(bin)
  Constant11/1 -> fir_next11/1(ain)
  Constant10/1 -> fir_next10/1(ain)
  fir_next8/2(pcout) -> fir_next9/3(pcin)
  fir_next8/1(bout) -> fir_next9/2(bin)
  Constant9/1 -> fir_next9/1(ain)
  fir_next7/2(pcout) -> fir_next8/3(pcin)
  fir_next7/1(bout) -> fir_next8/2(bin)
  Constant8/1 -> fir_next8/1(ain)
  fir_next5/2(pcout) -> fir_next6/3(pcin)
  fir_next5/1(bout) -> fir_next6/2(bin)
  fir_next6/2(pcout) -> fir_next7/3(pcin)
  fir_next6/1(bout) -> fir_next7/2(bin)
  Constant7/1 -> fir_next7/1(ain)
  Constant6/1 -> fir_next6/1(ain)
  fir_next4/2(pcout) -> fir_next5/3(pcin)
  fir_next4/1(bout) -> fir_next5/2(bin)
  Constant5/1 -> fir_next5/1(ain)
  fir_next2/2(pcout) -> fir_next3/3(pcin)
  fir_next2/1(bout) -> fir_next3/2(bin)
  fir_next3/2(pcout) -> fir_next4/3(pcin)
  fir_next3/1(bout) -> fir_next4/2(bin)
  Constant4/1 -> fir_next4/1(ain)
  Constant3/1 -> fir_next3/1(ain)
  fir_next1/2(pcout) -> fir_next2/3(pcin)
  fir_next1/1(bout) -> fir_next2/2(bin)
  Constant2/1 -> fir_next2/1(ain)
  fir_start/2(pcout) -> fir_next1/3(pcin)
  fir_start/1(bout) -> fir_next1/2(bin)
  Constant1/1 -> fir_next1/1(ain)
  Constant42/1 -> fir_start/1(ain)
  fir_last/1(p) -> out/1
  din/1 -> fir_start/2(bin)
  c/1 -> fir_start/3(c)

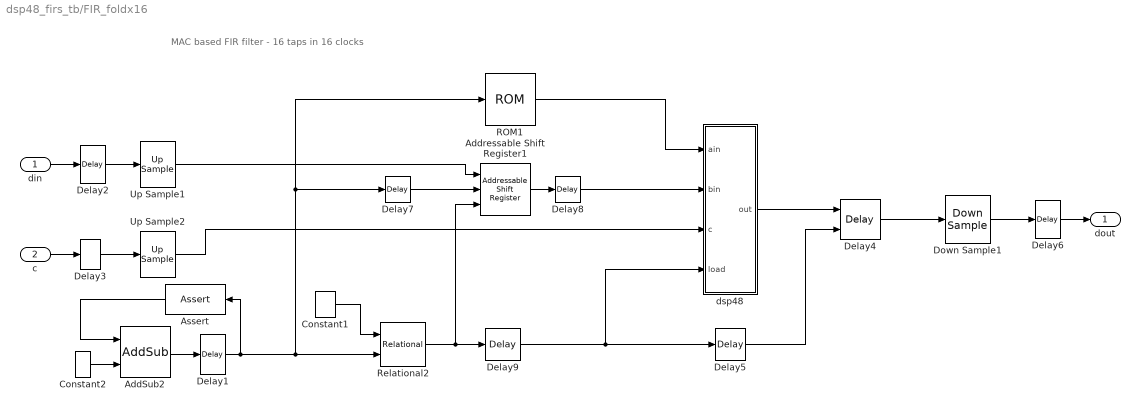
== system dsp48_firs_tb/FIR_foldx16 ==
  note: MAC based FIR filter - 16 taps in 16 clocks
  din : Inport  OutDataType=sfix(16)  OutScaling=2^0
  c : Inport  Port=2  OutDataType=sfix(16)  OutScaling=2^0
  AddSub2 : xbsIndex_r4/AddSub  mode=Addition  use_carryin=off  use_carryout=off  en=off  latency=0  precision=User Defined  arith_type=Unsigned  n_bits=4  bin_pt=0  quantization=Truncate  overflow=Wrap  dbl_ovrd=off  use_behavioral_HDL=off  pipelined=off  use_rpm=off  block_type=addsub
      settings: xl_area=[0, 0, 0, 0, 0, 0, 0]  block_version=VER_STRING_GOES_HERE
  Addressable Shift Register1 : xbsIndex_r4/Addressable Shift Register  infer_latency=on  depth=16  initVector=[0]  en=on  dbl_ovrd=off  use_behavioral_HDL=off  use_rpm=off  block_type=addrsr
      settings: infoedit="Delay of configurable length.  Any element in the delay line can be addressed and driven onto the output port.<P><P>Hardware notes: Implemented using SRL16s.  If a Virtex-II device is used, multiple SRLC16s are cascaded together."  xl_area=[0, 0, 0, 0, 0, 0, 0]  block_version=VER_STRING_GOES_HERE
  Assert : xbsIndex_r4/Assert  Orientation=left  assert_type=off  type_source=Explicitly  arith_type=Unsigned  n_bits=8  bin_pt=2  assert_rate=on  rate_source=Explicitly  period=1/16  output_port=on  block_type=assert
      settings: infoedit=Asserts a user-defined sample rate and/or type on a signal.  block_version=VER_STRING_GOES_HERE
  Constant1 : xbsIndex_r4/Constant  arith_type=Unsigned  const=0  n_bits=4  bin_pt=0  explicit_period=off  period=1  equ=P=C  opselect=C  inp2=PCIN>>17  opr=+  inp1=P  carry=CIN  dbl_ovrd=off  block_type=constant
      settings: block_version=VER_STRING_GOES_HERE
  Constant2 : xbsIndex_r4/Constant  arith_type=Unsigned  const=1  n_bits=4  bin_pt=0  explicit_period=off  period=1  equ=P=C  opselect=C  inp2=PCIN>>17  opr=+  inp1=P  carry=CIN  dbl_ovrd=off  block_type=constant
      settings: block_version=VER_STRING_GOES_HERE
  Delay{1..3,5..8} (7 alike) : xbsIndex_r4/Delay  en=off  latency=1  dbl_ovrd=off  reg_retiming=off  block_type=delay
      settings: infoedit="Delay line having  configurable length.<P><P>Hardware notes: A delay line is a chain, each link of which is an SRL16 followed by a flip-flop. If register retiming is enabled, the delay line is a chain of flip-flops."  xl_area=[0, 0, 0, 0, 0, 0, 0]  block_version=VER_STRING_GOES_HERE
  Delay4 : xbsIndex_r4/Delay  en=on  latency=1  dbl_ovrd=off  reg_retiming=off  block_type=delay
      settings: infoedit="Delay line having  configurable length.<P><P>Hardware notes: A delay line is a chain, each link of which is an SRL16 followed by a flip-flop. If register retiming is enabled, the delay line is a chain of flip-flops."  xl_area=[0, 0, 0, 0, 0, 0, 0]  block_version=VER_STRING_GOES_HERE
  Delay9 : xbsIndex_r4/Delay  en=off  latency=3  dbl_ovrd=off  reg_retiming=off  block_type=delay
      settings: infoedit="Delay line having  configurable length.<P><P>Hardware notes: A delay line is a chain, each link of which is an SRL16 followed by a flip-flop. If register retiming is enabled, the delay line is a chain of flip-flops."  xl_area=[0, 0, 0, 0, 0, 0, 0]  block_version=VER_STRING_GOES_HERE
  Down Sample1 : xbsIndex_r4/Down Sample  sample_ratio=16  sample_phase="Last Value of Frame  (most efficient)"  en=off  latency=1  dbl_ovrd=off  block_type=dsamp
      settings: xl_area=[0, 0, 0, 0, 0, 0, 0]  block_version=VER_STRING_GOES_HERE
  ROM1 : xbsIndex_r4/ROM  depth=16  initVector=coef(1:16)  distributed_mem=Distributed memory  rst=off  init_reg=0  en=off  latency=2  arith_type="Signed  (2's comp)"  n_bits=18  bin_pt=0  dbl_ovrd=off  optimize=Area  use_rpm=off  block_type=sprom
      settings: xl_area=[0, 0, 0, 0, 0, 0, 0]  block_version=VER_STRING_GOES_HERE
  Relational2 : xbsIndex_r4/Relational  mode=a=b  en=off  latency=0  dbl_ovrd=off  block_type=relational
      settings: xl_area=[0, 0, 0, 0, 0, 0, 0]  block_version=VER_STRING_GOES_HERE
  Up Sample1 : xbsIndex_r4/Up Sample  sample_ratio=16  copy_samples=on  dbl_ovrd=off  block_type=usamp
      settings: infoedit="Up samples input data.  Inserted values  can be zeros or copies of the most recent input sample.<P><P>Hardware notes: No hardware is needed if inserted values are copies of the input sample; otherwise, a mux and single bit flip-flop are used."  xl_area=[0, 0, 0, 0, 0, 0, 0]  block_version=VER_STRING_GOES_HERE
  Up Sample2 : xbsIndex_r4/Up Sample  sample_ratio=16  copy_samples=on  dbl_ovrd=off  block_type=usamp
      settings: infoedit="Up samples input data.  Inserted values  can be zeros or copies of the most recent input sample.<P><P>Hardware notes: No hardware is needed if inserted values are copies of the input sample; otherwise, a mux and single bit flip-flop are used."  xl_area=[0, 0, 0, 0, 0, 0, 0]  block_version=VER_STRING_GOES_HERE
  dsp48 : Subsystem
  dout : Outport  OutDataType=sfix(16)  OutScaling=2^0
  wires:
  Delay9/1 -> dsp48/4(load), Delay5/1
  Up Sample2/1 -> dsp48/3(c)
  Up Sample1/1 -> Addressable Shift Register1/1
  Delay4/1 -> Down Sample1/1
  Delay5/1 -> Delay4/2
  Constant1/1 -> Relational2/1
  Down Sample1/1 -> Delay6/1
  din/1 -> Delay2/1
  AddSub2/1 -> Delay1/1
  Constant2/1 -> AddSub2/2
  Delay2/1 -> Up Sample1/1
  Delay6/1 -> dout/1
  ROM1/1 -> dsp48/1(ain)
  dsp48/1(out) -> Delay4/1
  Addressable Shift Register1/1 -> Delay8/1
  c/1 -> Delay3/1
  Delay3/1 -> Up Sample2/1
  Delay1/1 -> Relational2/2, Delay7/1, ROM1/1, Assert/1
  Relational2/1 -> Delay9/1, Addressable Shift Register1/3
  Delay7/1 -> Addressable Shift Register1/2
  Delay8/1 -> dsp48/2(bin)
  Assert/1 -> AddSub2/1

== system dsp48_firs_tb/More Info ==

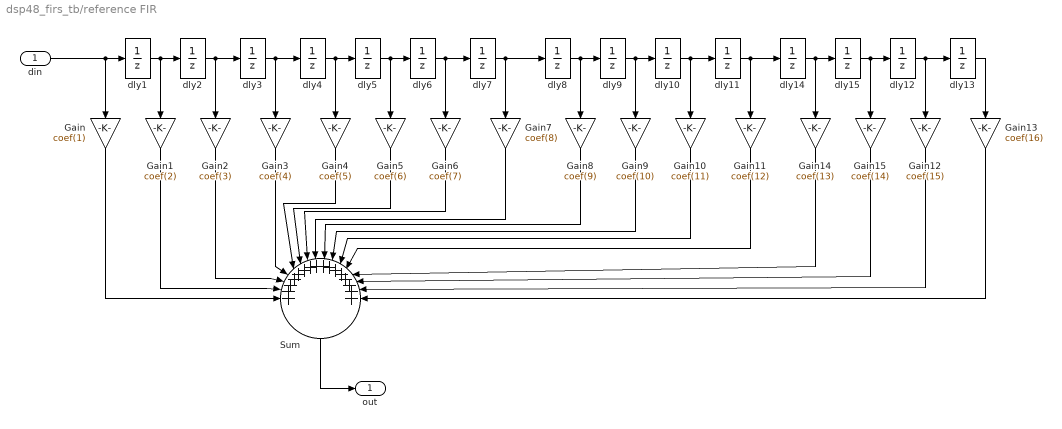
== system dsp48_firs_tb/reference FIR ==
  din : Inport  OutDataType=sfix(16)  OutScaling=2^0
  Gain : Gain  Orientation=down  Gain=coef(1)  ParameterDataType=sfix(16)  ParameterScaling=2^0  OutDataType=sfix(16)  OutScaling=2^0  SaturateOnIntegerOverflow=on
  Gain1 : Gain  Orientation=down  Gain=coef(2)  ParameterDataType=sfix(16)  ParameterScaling=2^0  OutDataType=sfix(16)  OutScaling=2^0  SaturateOnIntegerOverflow=on
  Gain10 : Gain  Orientation=down  Gain=coef(11)  ParameterDataType=sfix(16)  ParameterScaling=2^0  OutDataType=sfix(16)  OutScaling=2^0  SaturateOnIntegerOverflow=on
  Gain11 : Gain  Orientation=down  Gain=coef(12)  ParameterDataType=sfix(16)  ParameterScaling=2^0  OutDataType=sfix(16)  OutScaling=2^0  SaturateOnIntegerOverflow=on
  Gain12 : Gain  Orientation=down  Gain=coef(15)  ParameterDataType=sfix(16)  ParameterScaling=2^0  OutDataType=sfix(16)  OutScaling=2^0  SaturateOnIntegerOverflow=on
  Gain13 : Gain  Orientation=down  Gain=coef(16)  ParameterDataType=sfix(16)  ParameterScaling=2^0  OutDataType=sfix(16)  OutScaling=2^0  SaturateOnIntegerOverflow=on
  Gain14 : Gain  Orientation=down  Gain=coef(13)  ParameterDataType=sfix(16)  ParameterScaling=2^0  OutDataType=sfix(16)  OutScaling=2^0  SaturateOnIntegerOverflow=on
  Gain15 : Gain  Orientation=down  Gain=coef(14)  ParameterDataType=sfix(16)  ParameterScaling=2^0  OutDataType=sfix(16)  OutScaling=2^0  SaturateOnIntegerOverflow=on
  Gain2 : Gain  Orientation=down  Gain=coef(3)  ParameterDataType=sfix(16)  ParameterScaling=2^0  OutDataType=sfix(16)  OutScaling=2^0  SaturateOnIntegerOverflow=on
  Gain3 : Gain  Orientation=down  Gain=coef(4)  ParameterDataType=sfix(16)  ParameterScaling=2^0  OutDataType=sfix(16)  OutScaling=2^0  SaturateOnIntegerOverflow=on
  Gain4 : Gain  Orientation=down  Gain=coef(5)  ParameterDataType=sfix(16)  ParameterScaling=2^0  OutDataType=sfix(16)  OutScaling=2^0  SaturateOnIntegerOverflow=on
  Gain5 : Gain  Orientation=down  Gain=coef(6)  ParameterDataType=sfix(16)  ParameterScaling=2^0  OutDataType=sfix(16)  OutScaling=2^0  SaturateOnIntegerOverflow=on
  Gain6 : Gain  Orientation=down  Gain=coef(7)  ParameterDataType=sfix(16)  ParameterScaling=2^0  OutDataType=sfix(16)  OutScaling=2^0  SaturateOnIntegerOverflow=on
  Gain7 : Gain  Orientation=down  Gain=coef(8)  ParameterDataType=sfix(16)  ParameterScaling=2^0  OutDataType=sfix(16)  OutScaling=2^0  SaturateOnIntegerOverflow=on
  Gain8 : Gain  Orientation=down  Gain=coef(9)  ParameterDataType=sfix(16)  ParameterScaling=2^0  OutDataType=sfix(16)  OutScaling=2^0  SaturateOnIntegerOverflow=on
  Gain9 : Gain  Orientation=down  Gain=coef(10)  ParameterDataType=sfix(16)  ParameterScaling=2^0  OutDataType=sfix(16)  OutScaling=2^0  SaturateOnIntegerOverflow=on
  Sum : Sum  Orientation=down  Inputs=++++++++++++++++  OutDataType=sfix(16)  OutScaling=2^0  SaturateOnIntegerOverflow=on
  dly{1..15} (15 alike) : UnitDelay
  out : Outport  OutDataType=sfix(16)  OutScaling=2^0
  wires:
  din/1 -> dly1/1, Gain/1
  dly1/1 -> dly2/1, Gain1/1
  dly2/1 -> dly3/1, Gain2/1
  dly3/1 -> Gain3/1, dly4/1
  dly4/1 -> Gain4/1, dly5/1
  dly5/1 -> Gain5/1, dly6/1
  dly6/1 -> Gain6/1, dly7/1
  dly7/1 -> Gain7/1, dly8/1
  dly8/1 -> dly9/1, Gain8/1
  dly9/1 -> dly10/1, Gain9/1
  dly10/1 -> dly11/1, Gain10/1
  dly11/1 -> Gain11/1, dly14/1
  dly14/1 -> Gain14/1, dly15/1
  dly15/1 -> Gain15/1, dly12/1
  dly12/1 -> Gain12/1, dly13/1
  dly13/1 -> Gain13/1
  Gain/1 -> Sum/1
  Gain1/1 -> Sum/2
  Gain2/1 -> Sum/3
  Gain3/1 -> Sum/4
  Gain4/1 -> Sum/5
  Gain5/1 -> Sum/6
  Gain6/1 -> Sum/7
  Gain7/1 -> Sum/8
  Sum/1 -> out/1
  Gain8/1 -> Sum/9
  Gain9/1 -> Sum/10
  Gain10/1 -> Sum/11
  Gain11/1 -> Sum/12
  Gain14/1 -> Sum/13
  Gain15/1 -> Sum/14
  Gain12/1 -> Sum/15
  Gain13/1 -> Sum/16

== system dsp48_firs_tb/Basic C-MEX Template /Basic C-MEX Template  ==
